simulink model "Exp2_Model_RLC"  (R2023b)
settings: Solver=ode3  StartTime=0.0  StopTime=Time(end)  FixedStep=1e-6  RelTol=1e-3
undefined symbols (not defined in the file): den, num
settings Model: Creator=tunkarlu  LastModifiedBy=tunkarlu

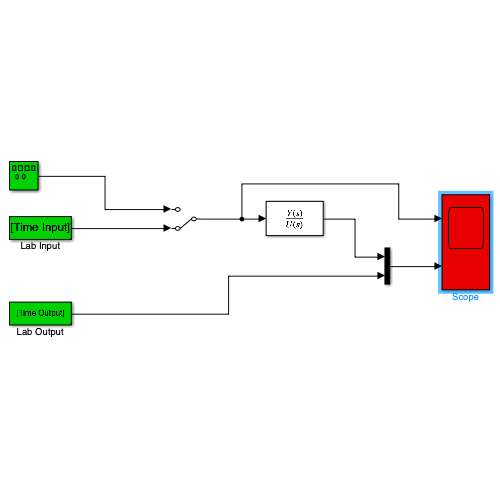
[thumbnail: Simulink's stored preview of the top-level diagram]
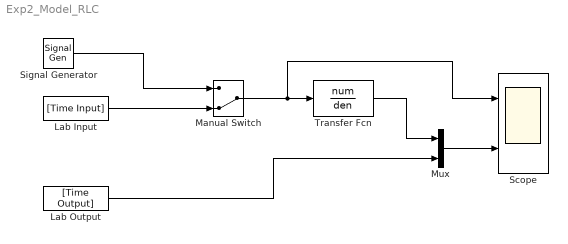
== system Exp2_Model_RLC ==
  Lab Input : FromWorkspace  VariableName=[Time Input]
  Lab Output : FromWorkspace  VariableName=[Time Output]
  Manual Switch : ManualSwitch  CurrentSetting=0
  Mux : Mux  Inputs=2
  Scope : Scope  NumInputPorts=2
  Signal Generator : SignalGenerator  WaveForm=square  Amplitude=3.149  Frequency=10
  Transfer Fcn : TransferFcn  Numerator=num  Denominator=den
  wires:
  Manual Switch/1 -> Scope/1, Transfer Fcn/1
  Lab Input/1 -> Manual Switch/2
  Signal Generator/1 -> Manual Switch/1
  Mux/1 -> Scope/2
  Transfer Fcn/1 -> Mux/1
  Lab Output/1 -> Mux/2
